simulink model "ultrason_model"  (R2013b)
settings: Solver=ode3  SolverMode=SingleTasking  StartTime=0.0  StopTime=inf  RelTol=1e-3
libraries: arduinolib x2
settings Model: SimulationMode=external  ExtModeTrigDuration=2  Creator=KOUSTA  LastModifiedBy=KOUSTA
settings OptimizationCC: OptimizeModelRefInitCode=on  LifeSpan=1
settings DebuggingCC: SolverPrmCheckMsg=none
settings HardwareCC: ProdBitPerInt=16  ProdBitPerPointer=8  ProdIntDivRoundTo=Zero  ProdEndianess=LittleEndian  ProdWordSize=8  ProdHWDeviceType=Atmel->AVR
settings RTWCC: SystemTargetFile=realtime.tlc  GenerateMakefile=off  TemplateMakefile=realtime.tmf  Description=Run on Target Hardware  RTWVerbose=off  ProcessScript=realtime_make_rtw_hook
settings STFCustomTargetCC: TargetLibSuffix=.a  GenerateSampleERTMain=on  ERTCustomFileBanners=on  SupportNonInlinedSFcns=off  SupportVariableSizeSignals=on  MATLABClassNameForMDSCustomization=Simulink.SoftwareTarget.ERTCustomization  GRTInterface=off  SystemTargetFile=realtime.tlc
settings ERTTargetCC: CodeReplacementLibrary=ANSI_C  GenerateSampleERTMain=on  ParMdlRefBuildCompliant=off  CompOptLevelCompliant=off  ConcurrentExecutionCompliant=off  CombineOutputUpdateFcns=off  ERTFirstTimeCompliant=off  SupportContinuousTime=on  SupportVariableSizeSignals=on  ModelStepFunctionPrototypeControlCompliant=off  CPPClassGenCompliant=off  ExtModeTransport=3  ExtModeMexFile=ext_serial_win32_comm  ExtModeMexArgs=0 1 9600  InlinedParameterPlacement=NonHierarchical  ERTSrcFileBannerTemplate=realtime_code_template.cgt  ERTHdrFileBannerTemplate=realtime_code_template.cgt  ERTDataSrcFileTemplate=realtime_code_template.cgt  ERTDataHdrFileTemplate=realtime_code_template.cgt  ERTCustomFileTemplate=realtime_file_process.tlc

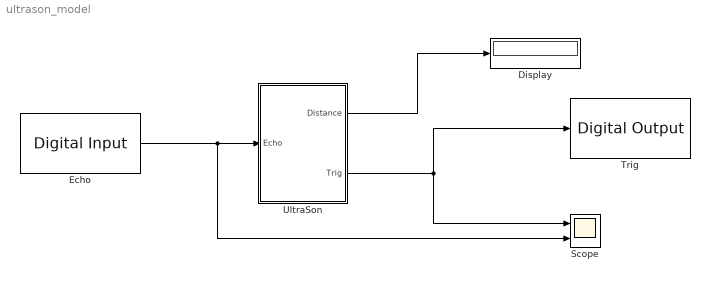
== system ultrason_model ==
  Display : Display
  Echo : arduinolib/Digital Input  pinNumber=11  sampleTime=1
  Scope : Scope  NumInputPorts=2
      settings: YMin=-5~-5  YMax=5~5
  Trig : arduinolib/Digital Output  pinNumber=12
  "UltraSon " : Subsystem
  wires:
  "UltraSon "/2(Trig) -> Trig/1, Scope/1
  Echo/1 -> Scope/2, "UltraSon "/1(Echo)
  "UltraSon "/1(Distance) -> Display/1

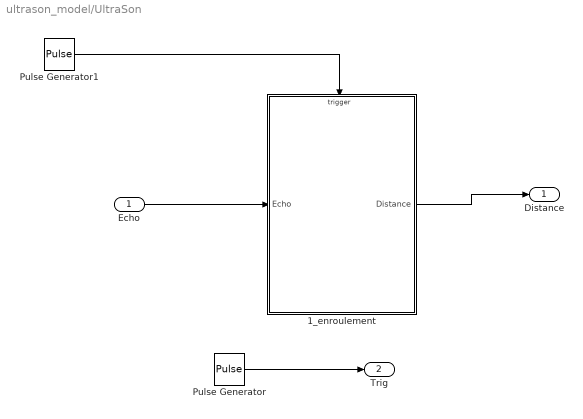
== system ultrason_model/UltraSon  ==
  Echo : Inport
  1_enroulement : Stateflow chart  TreatAsAtomicUnit=on
  Pulse Generator : DiscretePulseGenerator  PulseType=Time based  Period=1  PulseWidth=5
  Pulse Generator1 : DiscretePulseGenerator  PulseType=Time based  Period=10^(-6)  PulseWidth=5
  Distance : Outport
  Trig : Outport  Port=2
  wires:
  Echo/1 -> 1_enroulement/1(Echo)
  1_enroulement/1(Distance) -> Distance/1
  Pulse Generator/1 -> Trig/1
  Pulse Generator1/1 -> 1_enroulement/Trigger

== stateflow chart ultrason_model/UltraSon /1_enroulement ==
  state Etat0
    Q=0;
  state Etat2
    Distance=cont/55;
  state Etat1
    cont=cont+1;
  Etat0 -> Etat0 [order 2] : [!Echo]
  (default) -> Etat0
  Etat0 -> Etat1 [order 1] : [Echo]
  Etat2 -> Etat0
  Etat1 -> Etat2 [order 1] : [!Echo]
  Etat1 -> Etat1 [order 2] : [Echo]
  data: Echo input; Q local double; cont local double; Distance output double
  events: event input RISING_EDGE_EVENT
